simulink model "pitchangleacc"  (R2020a)
settings: Solver=VariableStepAuto  StartTime=0.0  StopTime=10.0  RelTol=1e-3
undefined symbols (not defined in the file): I, Ixx, Iyy, Izz, Jr
settings Model: Creator=Muni Kumar  LastModifiedBy=Muni Kumar

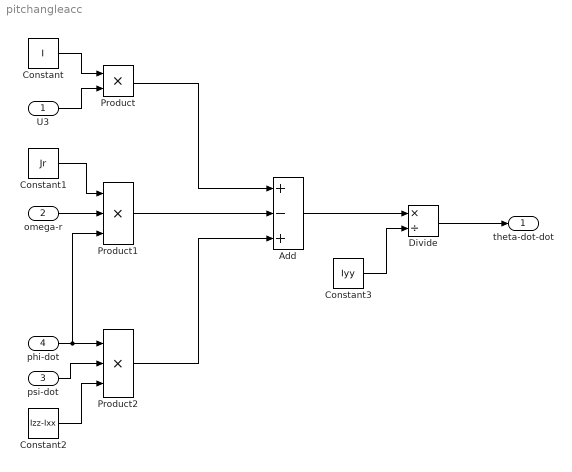
== system pitchangleacc ==
  U3 : Inport
  omega-r : Inport  Port=2
  psi-dot : Inport  Port=3
  phi-dot : Inport  Port=4
  Add : Sum  Inputs=+-+
  Constant : Constant  Value=I
  Constant1 : Constant  Value=Jr
  Constant2 : Constant  Value=Izz-Ixx
  Constant3 : Constant  Value=Iyy
  Divide : Product  Inputs=*/
  Product : Product
  Product1 : Product  Inputs=3
  Product2 : Product  Inputs=3
  theta-dot-dot : Outport
  wires:
  Divide/1 -> theta-dot-dot/1
  Constant1/1 -> Product1/1
  Product/1 -> Add/1
  Product2/1 -> Add/3
  Constant2/1 -> Product2/3
  Constant3/1 -> Divide/2
  omega-r/1 -> Product1/2
  Add/1 -> Divide/1
  Product1/1 -> Add/2
  psi-dot/1 -> Product2/2
  U3/1 -> Product/2
  Constant/1 -> Product/1
  phi-dot/1 -> Product1/3, Product2/1
